simulink model "LPL_Hopper_Model"  (R2023a)
settings: Solver=VariableStepAuto  StartTime=0.0  StopTime=10.0  RelTol=1e-3
settings Model: Creator=enson  LastModifiedBy=enson

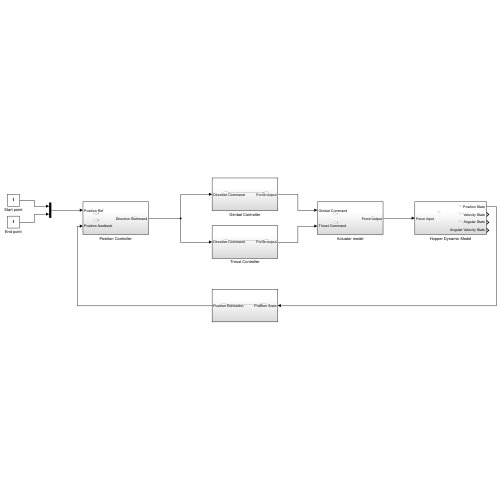
[thumbnail: Simulink's stored preview of the top-level diagram]
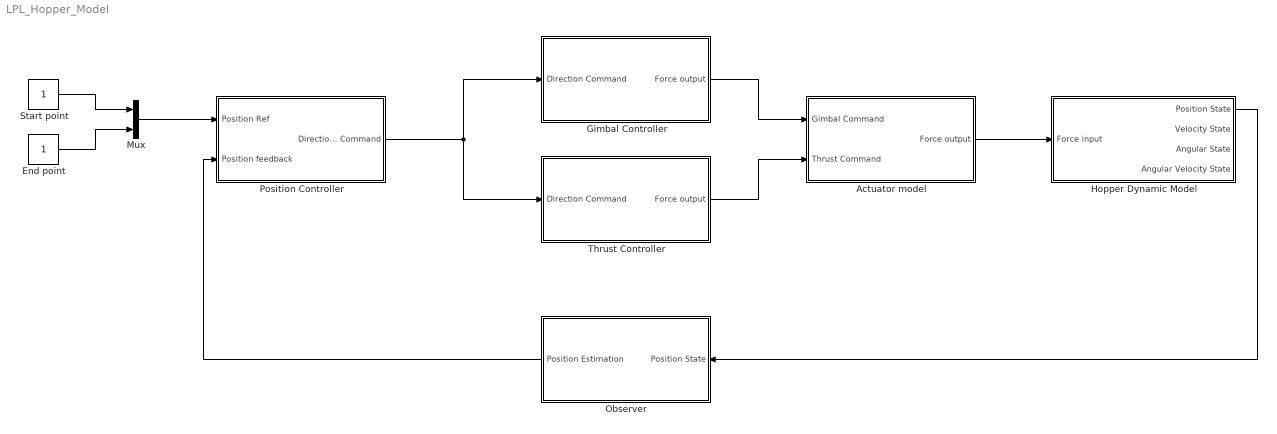
== system LPL_Hopper_Model ==
  Actuator model : Subsystem
  End point : Constant
  Gimbal Controller : Subsystem
  Hopper Dynamic Model : Subsystem
  Mux : Mux  Inputs=2
  Observer : Subsystem
  Position Controller : Subsystem
  Start point : Constant
  Thrust Controller : Subsystem
  wires:
  Mux/1 -> Position Controller/1(Position Ref)
  Start point/1 -> Mux/1
  End point/1 -> Mux/2
  Hopper Dynamic Model/1(Position State) -> Observer/1(Position State)
  Observer/1(Position Estimation) -> Position Controller/2(Position feedback)
  Position Controller/1(Direction Command) -> Gimbal Controller/1(Direction Command), Thrust Controller/1(Direction Command)
  Gimbal Controller/1(Force output) -> Actuator model/1(Gimbal Command)
  Thrust Controller/1(Force output) -> Actuator model/2(Thrust Command)
  Actuator model/1(Force output) -> Hopper Dynamic Model/1(Force input)

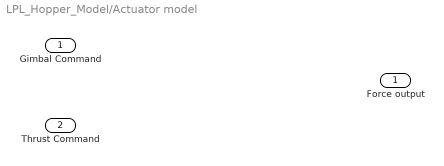
== system LPL_Hopper_Model/Actuator model ==
  Gimbal Command : Inport
  Thrust Command : Inport  Port=2
  Force output : Outport

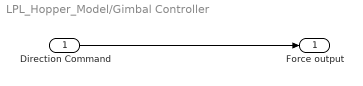
== system LPL_Hopper_Model/Gimbal Controller ==
  Direction Command : Inport
  Force output : Outport
  wires:
  Direction Command/1 -> Force output/1

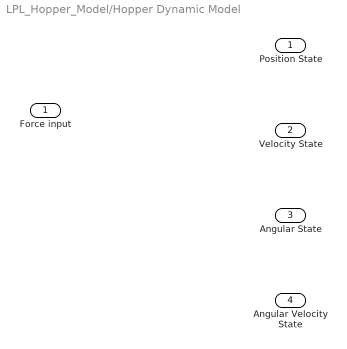
== system LPL_Hopper_Model/Hopper Dynamic Model ==
  Force input : Inport
  Position State : Outport
  Velocity State : Outport  Port=2
  Angular State : Outport  Port=3
  Angular Velocity State : Outport  Port=4

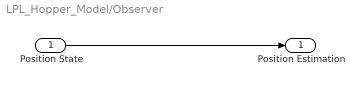
== system LPL_Hopper_Model/Observer ==
  Position State : Inport
  Position Estimation : Outport
  wires:
  Position State/1 -> Position Estimation/1

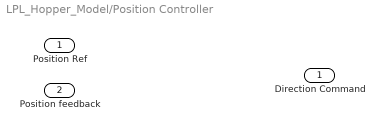
== system LPL_Hopper_Model/Position Controller ==
  Position Ref : Inport
  Position feedback : Inport  Port=2
  Direction Command : Outport

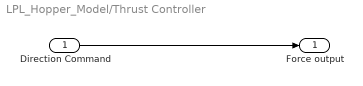
== system LPL_Hopper_Model/Thrust Controller ==
  Direction Command : Inport
  Force output : Outport
  wires:
  Direction Command/1 -> Force output/1
